simulink model "ES106A_StHlthSigStc"  (R2013b)
settings: Solver=FixedStepDiscrete  SolverMode=SingleTasking  StartTime=0.0  StopTime=1  FixedStep=0.002  RelTol=1e-3
undefined symbols (not defined in the file): APPL10_CNT_U08, BITSPERBYTE_CNT_U08, ENOTOK_CNT_U08, EOK_CNT_U08, LOWRMASKVAL_CNT_U32, NROFCRCAREA_CNT_U08, NVMAVRGPOSN_CNT_U08, NvmGetErrSts1, NVMMAXPOSN_CNT_U08, NVMMINPOSN_CNT_U08, NVMSAMPLECNTRPOSN_CNT_U08, RAMMAXPOSN_CNT_U08, RAMMINPOSN_CNT_U08, RAMRAWPOSN_CNT_U08, SIGCNT_ULS_U08, SigStcPrmInst, STHLTHMAXVAL_CNT_U08, STHLTHOSAPPL_CNT_U16, StHlthTaskRef1, WORDSIZE_CNT_U08
libraries: simulink x43, NxtrNvM x4, NxtrMax x4, NxtrMin x4, FloatToFixd x3, NxtrLim x2
(part 5 of 5)

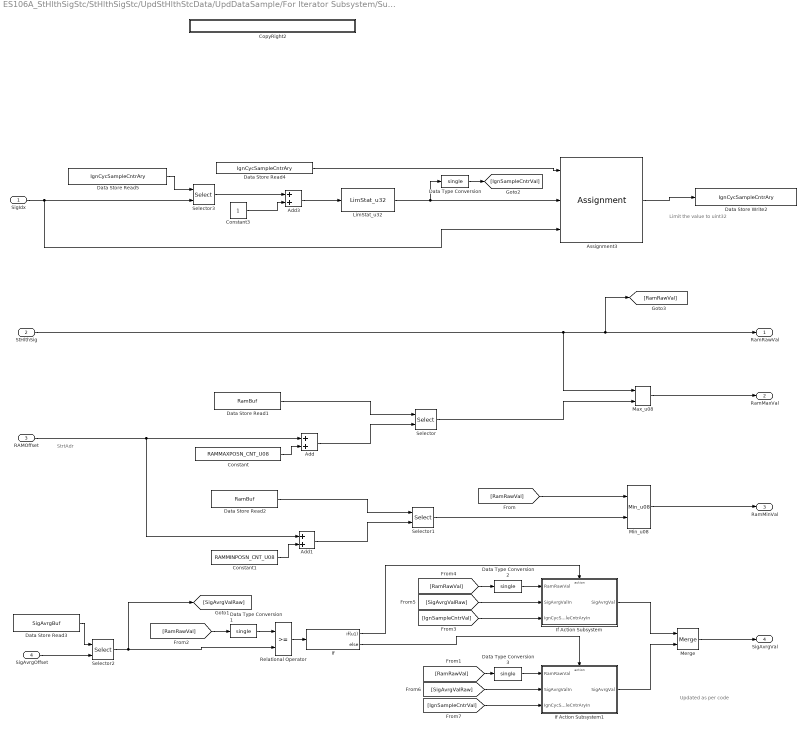
== system ES106A_StHlthSigStc/StHlthSigStc/UpdStHlthStcData/UpdDataSample/For Iterator Subsystem/Subsystem2/If Action Subsystem ==
  note: Updated as per code
  note: StrtAdr
  note: Limit the value to uint32
  SigIdx : Inport
  StHlthSig : Inport  Port=2
  RAMOffset : Inport  Port=3
  SigAvrgOffset : Inport  Port=4
  Add : Sum
  Add1 : Sum
  Add3 : Sum
  Assignment3 : Assignment  IndexMode=Zero-based  IndexOptions=Starting index (port)  Indices=1  OutputSizes=1
  Constant : Constant  Value=RAMMAXPOSN_CNT_U08  OutDataTypeStr=uint8
      settings: AttributesFormatString=%<OutDataTypeStr>
  Constant1 : Constant  Value=RAMMINPOSN_CNT_U08  OutDataTypeStr=uint8
      settings: AttributesFormatString=%<OutDataTypeStr>
  Constant3 : Constant  OutDataTypeStr=uint8
      settings: AttributesFormatString=%<OutDataTypeStr>
  CopyRight2 : Subsystem  Description=|  mask(Copyright Information){none=on}
      | Copyright info block.                                               
      |                                                                     
      | Place copyright information at the top of every subsystem in design.
      mask prompts: none "No parameters"
      mask help: Place copyright information at the top of every subsystem in design.
      mask Display:
      | NxtrConf = 'Nexteer Confidential';
      | 
      | sys = bdroot; %handle for the current model ("system")
      | first = get_param(sys,'Created');
      | first = first(end-3:end);  %year is last four digits
      | 
      | last = get_param(sys,'LastModifiedDate');
      | if isempty(last)
      |     last = datestr(now,'yyyy');
      | else
      |     last = last(end-3:end);
      | end
      | 
      | if strcmp(first,last)
      |     fprintf('%s -- Copyright %s Nexteer',NxtrConf,first)
      | else
      |     fprintf('%s -- %s%s- %s Nexteer',NxtrConf,char(169),first,last)
      | end
  Data Store Read1 : DataStoreRead  DataStoreName=RamBuf
  Data Store Read2 : DataStoreRead  DataStoreName=RamBuf
  Data Store Read3 : DataStoreRead  DataStoreName=SigAvrgBuf
  Data Store Read4 : DataStoreRead  Priority=2  DataStoreName=IgnCycSampleCntrAry
      settings: AttributesFormatString=Priority: %<Priority>
  Data Store Read5 : DataStoreRead  Priority=1  DataStoreName=IgnCycSampleCntrAry
      settings: AttributesFormatString=Priority: %<Priority>
  Data Store Write2 : DataStoreWrite  Priority=3  DataStoreName=IgnCycSampleCntrAry
      settings: AttributesFormatString=Priority: %<Priority>
  Data Type Conversion{,1..3} (4 alike) : DataTypeConversion  OutDataTypeStr=single
  If : If  IfExpression=u1
  If Action Subsystem : Subsystem  TreatAsAtomicUnit=on
  If Action Subsystem1 : Subsystem  TreatAsAtomicUnit=on
  LimStat_u32 : NxtrLim/LimStat_u32  LoLim=IGNCYCSAMPLECNTRARYMINLIM_CNT_U32  HiLim=IGNCYCSAMPLECNTRARYMAXLIM_CNT_U32
      settings: AttributesFormatString=|
      | Low Limit: %<LoLim>
      | High Limit:%<HiLim>
  Max_u08 : NxtrMax/Max_u08  SFunctionSpec="uint8 y1 = Max_u08( uint8 u1,  uint8 u2)"
      settings: AttributesFormatString=%<Name>
  Merge : Merge
  Min_u08 : NxtrMin/Min_u08  SFunctionSpec="uint8 y1 = Min_u08( uint8 u1,  uint8 u2)"  ShowSpec=off
      settings: AttributesFormatString=%<Name>
  Relational Operator : RelationalOperator  OutDataTypeStr=boolean
  Selector : Selector  IndexMode=Zero-based  InputPortWidth=66  IndexOptions=Starting index (port)  Indices=[1 3]  OutputSizes=1
  Selector1 : Selector  IndexMode=Zero-based  InputPortWidth=66  IndexOptions=Starting index (port)  Indices=[1 3]  OutputSizes=1
  Selector2 : Selector  IndexMode=Zero-based  InputPortWidth=22  IndexOptions=Starting index (port)  Indices=[1 3]  OutputSizes=1
  Selector3 : Selector  IndexMode=Zero-based  InputPortWidth=22  IndexOptions=Starting index (port)  Indices=[1 3]  OutputSizes=1
  RamRawVal : Outport
  RamMaxVal : Outport  Port=2
  RamMinVal : Outport  Port=3
  SigAvrgVal : Outport  Port=4
  wires:
  Data Store Read1/1 -> Selector/1
  Constant/1 -> Add/2
  Add/1 -> Selector/2
  Selector/1 -> Max_u08/2
  Data Store Read2/1 -> Selector1/1
  Constant1/1 -> Add1/2
  Add1/1 -> Selector1/2
  Selector1/1 -> Min_u08/2
  Data Store Read3/1 -> Selector2/1
  RAMOffset/1 -> Add1/1, Add/1
  Max_u08/1 -> RamMaxVal/1
  [RamRawVal] -> Min_u08/1
  Min_u08/1 -> RamMinVal/1
  Relational Operator/1 -> If/1
  If/1 -> If Action Subsystem/Action
  If/2 -> If Action Subsystem1/Action
  Merge/1 -> SigAvrgVal/1
  If Action Subsystem/1(SigAvrgVal) -> Merge/1
  If Action Subsystem1/1(SigAvrgVal) -> Merge/2
  [IgnSampleCntrVal] -> If Action Subsystem/3(IgnCycSampleCntrAryIn)
  SigAvrgOffset/1 -> Selector2/2
  [SigAvrgValRaw] -> If Action Subsystem1/2(SigAvrgValIn)
  [SigAvrgValRaw] -> If Action Subsystem/2(SigAvrgValIn)
  Selector2/1 -> Relational Operator/2, [SigAvrgValRaw]
  [RamRawVal] -> Data Type Conversion2/1
  [RamRawVal] -> Data Type Conversion3/1
  [RamRawVal] -> Data Type Conversion1/1
  Data Store Read5/1 -> Selector3/1
  Selector3/1 -> Add3/1
  Constant3/1 -> Add3/2
  Assignment3/1 -> Data Store Write2/1
  Add3/1 -> LimStat_u32/1
  Data Store Read4/1 -> Assignment3/1
  SigIdx/1 -> Assignment3/3, Selector3/2
  LimStat_u32/1 -> Data Type Conversion/1, Assignment3/2
  Data Type Conversion/1 -> [IgnSampleCntrVal]
  [IgnSampleCntrVal] -> If Action Subsystem1/3(IgnCycSampleCntrAryIn)
  StHlthSig/1 -> [RamRawVal], RamRawVal/1, Max_u08/1
  Data Type Conversion1/1 -> Relational Operator/1
  Data Type Conversion2/1 -> If Action Subsystem/1(RamRawVal)
  Data Type Conversion3/1 -> If Action Subsystem1/1(RamRawVal)

== system ES106A_StHlthSigStc/StHlthSigStc/UpdStHlthStcData/UpdDataSample/For Iterator Subsystem/Subsystem2/UpdateRamBuf ==
  note: RamAvrgVal Input was deleted
  RAMLocation : Inport
  RamRawVal : Inport  Port=2
  RamMaxVal : Inport  Port=3
  RamMinVal : Inport  Port=4
  Assignment4 : Assignment  IndexMode=Zero-based  IndexOptions=Starting index (port)  Indices=1  OutputSizes=1
  CopyRight2 : Subsystem  Description=|  mask(Copyright Information){none=on}
      | Copyright info block.                                               
      |                                                                     
      | Place copyright information at the top of every subsystem in design.
      mask prompts: none "No parameters"
      mask help: Place copyright information at the top of every subsystem in design.
      mask Display:
      | NxtrConf = 'Nexteer Confidential';
      | 
      | sys = bdroot; %handle for the current model ("system")
      | first = get_param(sys,'Created');
      | first = first(end-3:end);  %year is last four digits
      | 
      | last = get_param(sys,'LastModifiedDate');
      | if isempty(last)
      |     last = datestr(now,'yyyy');
      | else
      |     last = last(end-3:end);
      | end
      | 
      | if strcmp(first,last)
      |     fprintf('%s -- Copyright %s Nexteer',NxtrConf,first)
      | else
      |     fprintf('%s -- %s%s- %s Nexteer',NxtrConf,char(169),first,last)
      | end
  Data Store Read1 : DataStoreRead  DataStoreName=RamBuf
  Data Store Write2 : DataStoreWrite  DataStoreName=RamBuf
  Mux : Mux  Inputs=3
  wires:
  Data Store Read1/1 -> Assignment4/1
  RAMLocation/1 -> Assignment4/3
  Mux/1 -> Assignment4/2
  Assignment4/1 -> Data Store Write2/1
  RamRawVal/1 -> Mux/1
  RamMaxVal/1 -> Mux/2
  RamMinVal/1 -> Mux/3

== system ES106A_StHlthSigStc/StHlthSigStc/UpdStHlthStcData/UpdDataSample/For Iterator Subsystem/Subsystem2/UpdateSigAvrgBuf ==
  SigAvrgLocation : Inport
  SigAvrgVal : Inport  Port=2
  Assignment4 : Assignment  IndexMode=Zero-based  IndexOptions=Starting index (port)  Indices=1  OutputSizes=1
  CopyRight2 : Subsystem  Description=|  mask(Copyright Information){none=on}
      | Copyright info block.                                               
      |                                                                     
      | Place copyright information at the top of every subsystem in design.
      mask prompts: none "No parameters"
      mask help: Place copyright information at the top of every subsystem in design.
      mask Display:
      | NxtrConf = 'Nexteer Confidential';
      | 
      | sys = bdroot; %handle for the current model ("system")
      | first = get_param(sys,'Created');
      | first = first(end-3:end);  %year is last four digits
      | 
      | last = get_param(sys,'LastModifiedDate');
      | if isempty(last)
      |     last = datestr(now,'yyyy');
      | else
      |     last = last(end-3:end);
      | end
      | 
      | if strcmp(first,last)
      |     fprintf('%s -- Copyright %s Nexteer',NxtrConf,first)
      | else
      |     fprintf('%s -- %s%s- %s Nexteer',NxtrConf,char(169),first,last)
      | end
  Data Store Read1 : DataStoreRead  DataStoreName=SigAvrgBuf
  Data Store Write2 : DataStoreWrite  DataStoreName=SigAvrgBuf
  wires:
  Data Store Read1/1 -> Assignment4/1
  SigAvrgLocation/1 -> Assignment4/3
  Assignment4/1 -> Data Store Write2/1
  SigAvrgVal/1 -> Assignment4/2

== system ES106A_StHlthSigStc/StHlthSigStc/GetSigStcHlthData/If Action Subsystem1/GetSigStcHlthData/If Action Subsystem/While Iterator Subsystem/CopyRight2 ==

== system ES106A_StHlthSigStc/StHlthSigStc/GetSigStcHlthData/If Action Subsystem1/GetSigStcHlthData/If Action Subsystem/While Iterator Subsystem/Switch Case Action Subsystem ==
  In1 : Inport
  Action Port : ActionPort  ActionType=case
  CopyRight2 : Subsystem  Description=|  mask(Copyright Information){none=on}
      | Copyright info block.                                               
      |                                                                     
      | Place copyright information at the top of every subsystem in design.
      mask prompts: none "No parameters"
      mask help: Place copyright information at the top of every subsystem in design.
      mask Display:
      | NxtrConf = 'Nexteer Confidential';
      | 
      | sys = bdroot; %handle for the current model ("system")
      | first = get_param(sys,'Created');
      | if(isempty(first))
      |     first = datestr(now,'yyyy');
      | else
      |     first = first(end-3:end);  %year is last four digits
      | end
      | 
      | last = get_param(sys,'LastModifiedDate');
      | if isempty(last)
      |     last = datestr(now,'yyyy');
      | else
      |     last = last(end-3:end);
      | end
      | 
      | if strcmp(first,last)
      |     fprintf('%s -- Copyright %s Nexteer',NxtrConf,first)
      | else
      |     fprintf('%s -- %s%s- %s Nexteer',NxtrConf,char(169),first,last)
      | end
  Data Type Conversion : DataTypeConversion  OutDataTypeStr=uint32
  Shift Arithmetic3 : ArithShift  BitShiftNumber=SHIFTFAC24_ULS_U08  BitShiftDirection=Left
  Out1 : Outport
  wires:
  In1/1 -> Data Type Conversion/1
  Data Type Conversion/1 -> Shift Arithmetic3/1
  Shift Arithmetic3/1 -> Out1/1

== system ES106A_StHlthSigStc/StHlthSigStc/GetSigStcHlthData/If Action Subsystem1/GetSigStcHlthData/If Action Subsystem/While Iterator Subsystem/Switch Case Action Subsystem1 ==
  In1 : Inport
  Action Port : ActionPort  ActionType=case
  CopyRight2 : Subsystem  Description=|  mask(Copyright Information){none=on}
      | Copyright info block.                                               
      |                                                                     
      | Place copyright information at the top of every subsystem in design.
      mask prompts: none "No parameters"
      mask help: Place copyright information at the top of every subsystem in design.
      mask Display:
      | NxtrConf = 'Nexteer Confidential';
      | 
      | sys = bdroot; %handle for the current model ("system")
      | first = get_param(sys,'Created');
      | if(isempty(first))
      |     first = datestr(now,'yyyy');
      | else
      |     first = first(end-3:end);  %year is last four digits
      | end
      | 
      | last = get_param(sys,'LastModifiedDate');
      | if isempty(last)
      |     last = datestr(now,'yyyy');
      | else
      |     last = last(end-3:end);
      | end
      | 
      | if strcmp(first,last)
      |     fprintf('%s -- Copyright %s Nexteer',NxtrConf,first)
      | else
      |     fprintf('%s -- %s%s- %s Nexteer',NxtrConf,char(169),first,last)
      | end
  Data Type Conversion1 : DataTypeConversion  OutDataTypeStr=uint32
  Shift Arithmetic1 : ArithShift  BitShiftNumber=SHIFTFAC16_ULS_U08  BitShiftDirection=Left
  Out1 : Outport
  wires:
  In1/1 -> Data Type Conversion1/1
  Shift Arithmetic1/1 -> Out1/1
  Data Type Conversion1/1 -> Shift Arithmetic1/1

== system ES106A_StHlthSigStc/StHlthSigStc/GetSigStcHlthData/If Action Subsystem1/GetSigStcHlthData/If Action Subsystem/While Iterator Subsystem/Switch Case Action Subsystem2 ==
  In1 : Inport
  Action Port : ActionPort  ActionType=case
  CopyRight2 : Subsystem  Description=|  mask(Copyright Information){none=on}
      | Copyright info block.                                               
      |                                                                     
      | Place copyright information at the top of every subsystem in design.
      mask prompts: none "No parameters"
      mask help: Place copyright information at the top of every subsystem in design.
      mask Display:
      | NxtrConf = 'Nexteer Confidential';
      | 
      | sys = bdroot; %handle for the current model ("system")
      | first = get_param(sys,'Created');
      | if(isempty(first))
      |     first = datestr(now,'yyyy');
      | else
      |     first = first(end-3:end);  %year is last four digits
      | end
      | 
      | last = get_param(sys,'LastModifiedDate');
      | if isempty(last)
      |     last = datestr(now,'yyyy');
      | else
      |     last = last(end-3:end);
      | end
      | 
      | if strcmp(first,last)
      |     fprintf('%s -- Copyright %s Nexteer',NxtrConf,first)
      | else
      |     fprintf('%s -- %s%s- %s Nexteer',NxtrConf,char(169),first,last)
      | end
  Data Type Conversion1 : DataTypeConversion  OutDataTypeStr=uint32
  Shift Arithmetic2 : ArithShift  BitShiftNumber=SHIFTFAC8_ULS_U08  BitShiftDirection=Left
  Out1 : Outport
  wires:
  In1/1 -> Data Type Conversion1/1
  Data Type Conversion1/1 -> Shift Arithmetic2/1
  Shift Arithmetic2/1 -> Out1/1

== system ES106A_StHlthSigStc/StHlthSigStc/GetSigStcHlthData/If Action Subsystem1/GetSigStcHlthData/If Action Subsystem/While Iterator Subsystem/Switch Case Action Subsystem3 ==
  In1 : Inport
  Action Port : ActionPort  ActionType=case
  CopyRight2 : Subsystem  Description=|  mask(Copyright Information){none=on}
      | Copyright info block.                                               
      |                                                                     
      | Place copyright information at the top of every subsystem in design.
      mask prompts: none "No parameters"
      mask help: Place copyright information at the top of every subsystem in design.
      mask Display:
      | NxtrConf = 'Nexteer Confidential';
      | 
      | sys = bdroot; %handle for the current model ("system")
      | first = get_param(sys,'Created');
      | if(isempty(first))
      |     first = datestr(now,'yyyy');
      | else
      |     first = first(end-3:end);  %year is last four digits
      | end
      | 
      | last = get_param(sys,'LastModifiedDate');
      | if isempty(last)
      |     last = datestr(now,'yyyy');
      | else
      |     last = last(end-3:end);
      | end
      | 
      | if strcmp(first,last)
      |     fprintf('%s -- Copyright %s Nexteer',NxtrConf,first)
      | else
      |     fprintf('%s -- %s%s- %s Nexteer',NxtrConf,char(169),first,last)
      | end
  Data Type Conversion1 : DataTypeConversion  OutDataTypeStr=uint32
  Out1 : Outport
  wires:
  In1/1 -> Data Type Conversion1/1
  Data Type Conversion1/1 -> Out1/1

== system ES106A_StHlthSigStc/StHlthSigStc/StHlthStcPwrDwn/For Iterator Subsystem/If Action Subsystem/Statistical data computation for Controller Life Cycle/While Iterator Subsystem/CopyRight2 ==

== system ES106A_StHlthSigStc/StHlthSigStc/StHlthStcPwrDwn/For Iterator Subsystem/If Action Subsystem/Statistical data computation for Controller Life Cycle/While Iterator Subsystem/Switch Case Action Subsystem ==
  In1 : Inport
  Action Port : ActionPort  ActionType=case
  CopyRight2 : Subsystem  Description=|  mask(Copyright Information){none=on}
      | Copyright info block.                                               
      |                                                                     
      | Place copyright information at the top of every subsystem in design.
      mask prompts: none "No parameters"
      mask help: Place copyright information at the top of every subsystem in design.
      mask Display:
      | NxtrConf = 'Nexteer Confidential';
      | 
      | sys = bdroot; %handle for the current model ("system")
      | first = get_param(sys,'Created');
      | if(isempty(first))
      |     first = datestr(now,'yyyy');
      | else
      |     first = first(end-3:end);  %year is last four digits
      | end
      | 
      | last = get_param(sys,'LastModifiedDate');
      | if isempty(last)
      |     last = datestr(now,'yyyy');
      | else
      |     last = last(end-3:end);
      | end
      | 
      | if strcmp(first,last)
      |     fprintf('%s -- Copyright %s Nexteer',NxtrConf,first)
      | else
      |     fprintf('%s -- %s%s- %s Nexteer',NxtrConf,char(169),first,last)
      | end
  Data Type Conversion : DataTypeConversion  OutDataTypeStr=uint32
  Shift Arithmetic3 : ArithShift  BitShiftNumber=SHIFTFAC24_ULS_U08  BitShiftDirection=Left
  Out1 : Outport
  wires:
  In1/1 -> Data Type Conversion/1
  Data Type Conversion/1 -> Shift Arithmetic3/1
  Shift Arithmetic3/1 -> Out1/1

== system ES106A_StHlthSigStc/StHlthSigStc/StHlthStcPwrDwn/For Iterator Subsystem/If Action Subsystem/Statistical data computation for Controller Life Cycle/While Iterator Subsystem/Switch Case Action Subsystem1 ==
  In1 : Inport
  Action Port : ActionPort  ActionType=case
  CopyRight2 : Subsystem  Description=|  mask(Copyright Information){none=on}
      | Copyright info block.                                               
      |                                                                     
      | Place copyright information at the top of every subsystem in design.
      mask prompts: none "No parameters"
      mask help: Place copyright information at the top of every subsystem in design.
      mask Display:
      | NxtrConf = 'Nexteer Confidential';
      | 
      | sys = bdroot; %handle for the current model ("system")
      | first = get_param(sys,'Created');
      | if(isempty(first))
      |     first = datestr(now,'yyyy');
      | else
      |     first = first(end-3:end);  %year is last four digits
      | end
      | 
      | last = get_param(sys,'LastModifiedDate');
      | if isempty(last)
      |     last = datestr(now,'yyyy');
      | else
      |     last = last(end-3:end);
      | end
      | 
      | if strcmp(first,last)
      |     fprintf('%s -- Copyright %s Nexteer',NxtrConf,first)
      | else
      |     fprintf('%s -- %s%s- %s Nexteer',NxtrConf,char(169),first,last)
      | end
  Data Type Conversion1 : DataTypeConversion  OutDataTypeStr=uint32
  Shift Arithmetic1 : ArithShift  BitShiftNumber=SHIFTFAC16_ULS_U08  BitShiftDirection=Left
  Out1 : Outport
  wires:
  In1/1 -> Data Type Conversion1/1
  Shift Arithmetic1/1 -> Out1/1
  Data Type Conversion1/1 -> Shift Arithmetic1/1

== system ES106A_StHlthSigStc/StHlthSigStc/StHlthStcPwrDwn/For Iterator Subsystem/If Action Subsystem/Statistical data computation for Controller Life Cycle/While Iterator Subsystem/Switch Case Action Subsystem2 ==
  In1 : Inport
  Action Port : ActionPort  ActionType=case
  CopyRight2 : Subsystem  Description=|  mask(Copyright Information){none=on}
      | Copyright info block.                                               
      |                                                                     
      | Place copyright information at the top of every subsystem in design.
      mask prompts: none "No parameters"
      mask help: Place copyright information at the top of every subsystem in design.
      mask Display:
      | NxtrConf = 'Nexteer Confidential';
      | 
      | sys = bdroot; %handle for the current model ("system")
      | first = get_param(sys,'Created');
      | if(isempty(first))
      |     first = datestr(now,'yyyy');
      | else
      |     first = first(end-3:end);  %year is last four digits
      | end
      | 
      | last = get_param(sys,'LastModifiedDate');
      | if isempty(last)
      |     last = datestr(now,'yyyy');
      | else
      |     last = last(end-3:end);
      | end
      | 
      | if strcmp(first,last)
      |     fprintf('%s -- Copyright %s Nexteer',NxtrConf,first)
      | else
      |     fprintf('%s -- %s%s- %s Nexteer',NxtrConf,char(169),first,last)
      | end
  Data Type Conversion1 : DataTypeConversion  OutDataTypeStr=uint32
  Shift Arithmetic2 : ArithShift  BitShiftNumber=SHIFTFAC8_ULS_U08  BitShiftDirection=Left
  Out1 : Outport
  wires:
  In1/1 -> Data Type Conversion1/1
  Data Type Conversion1/1 -> Shift Arithmetic2/1
  Shift Arithmetic2/1 -> Out1/1

== system ES106A_StHlthSigStc/StHlthSigStc/StHlthStcPwrDwn/For Iterator Subsystem/If Action Subsystem/Statistical data computation for Controller Life Cycle/While Iterator Subsystem/Switch Case Action Subsystem3 ==
  In1 : Inport
  Action Port : ActionPort  ActionType=case
  CopyRight2 : Subsystem  Description=|  mask(Copyright Information){none=on}
      | Copyright info block.                                               
      |                                                                     
      | Place copyright information at the top of every subsystem in design.
      mask prompts: none "No parameters"
      mask help: Place copyright information at the top of every subsystem in design.
      mask Display:
      | NxtrConf = 'Nexteer Confidential';
      | 
      | sys = bdroot; %handle for the current model ("system")
      | first = get_param(sys,'Created');
      | if(isempty(first))
      |     first = datestr(now,'yyyy');
      | else
      |     first = first(end-3:end);  %year is last four digits
      | end
      | 
      | last = get_param(sys,'LastModifiedDate');
      | if isempty(last)
      |     last = datestr(now,'yyyy');
      | else
      |     last = last(end-3:end);
      | end
      | 
      | if strcmp(first,last)
      |     fprintf('%s -- Copyright %s Nexteer',NxtrConf,first)
      | else
      |     fprintf('%s -- %s%s- %s Nexteer',NxtrConf,char(169),first,last)
      | end
  Data Type Conversion1 : DataTypeConversion  OutDataTypeStr=uint32
  Out1 : Outport
  wires:
  In1/1 -> Data Type Conversion1/1
  Data Type Conversion1/1 -> Out1/1

== system ES106A_StHlthSigStc/StHlthSigStc/StHlthStcPwrDwn/For Iterator Subsystem/If Action Subsystem/Update Nvm/Subsystem/CopyRight2 ==

== system ES106A_StHlthSigStc/StHlthSigStc/StHlthStcPwrDwn/For Iterator Subsystem/If Action Subsystem/Update Nvm/Subsystem1/CopyRight2 ==

== system ES106A_StHlthSigStc/StHlthSigStc/UpdStHlthStcData/Call Non Trusted Function /For Iterator Subsystem/Subsystem2/If Action Subsystem/CopyRight2 ==

== system ES106A_StHlthSigStc/StHlthSigStc/UpdStHlthStcData/Call Non Trusted Function /For Iterator Subsystem/Subsystem2/If Action Subsystem/If Action Subsystem ==
  RamRawVal : Inport
  SigAvrgValIn : Inport  Port=2
  IgnCycSampleCntrAryIn : Inport  Port=3
  Action Port : ActionPort  ActionType=then
  Add1 : Sum
  Add4 : Sum  Inputs=+-
  Divide : Product  Inputs=*/
  SigAvrgVal : Outport
  wires:
  [SigAvrgVal] -> Add4/2
  RamRawVal/1 -> Add4/1
  Add4/1 -> Divide/1
  IgnCycSampleCntrAryIn/1 -> Divide/2
  SigAvrgValIn/1 -> [SigAvrgVal]
  Divide/1 -> Add1/2
  [SigAvrgVal] -> Add1/1
  Add1/1 -> SigAvrgVal/1

== system ES106A_StHlthSigStc/StHlthSigStc/UpdStHlthStcData/Call Non Trusted Function /For Iterator Subsystem/Subsystem2/If Action Subsystem/If Action Subsystem1 ==
  RamRawVal : Inport
  SigAvrgValIn : Inport  Port=2
  IgnCycSampleCntrAryIn : Inport  Port=3
  Action Port : ActionPort  ActionType=else
  Add1 : Sum  Inputs=+-
  Add4 : Sum  Inputs=+-
  Divide : Product  Inputs=*/
  SigAvrgVal : Outport
  wires:
  RamRawVal/1 -> Add4/2
  Add4/1 -> Divide/1
  IgnCycSampleCntrAryIn/1 -> Divide/2
  SigAvrgValIn/1 -> [SigAvrgVal]
  Divide/1 -> Add1/2
  [SigAvrgVal] -> Add1/1
  Add1/1 -> SigAvrgVal/1
  [SigAvrgVal] -> Add4/1

== system ES106A_StHlthSigStc/StHlthSigStc/UpdStHlthStcData/Call Non Trusted Function /For Iterator Subsystem/Subsystem2/UpdateRamBuf/CopyRight2 ==

== system ES106A_StHlthSigStc/StHlthSigStc/UpdStHlthStcData/Call Non Trusted Function /For Iterator Subsystem/Subsystem2/UpdateSigAvrgBuf/CopyRight2 ==

== system ES106A_StHlthSigStc/StHlthSigStc/UpdStHlthStcData/UpdDataSample/For Iterator Subsystem/Subsystem2/If Action Subsystem/CopyRight2 ==

== system ES106A_StHlthSigStc/StHlthSigStc/UpdStHlthStcData/UpdDataSample/For Iterator Subsystem/Subsystem2/If Action Subsystem/If Action Subsystem ==
  RamRawVal : Inport
  SigAvrgValIn : Inport  Port=2
  IgnCycSampleCntrAryIn : Inport  Port=3
  Action Port : ActionPort  ActionType=then
  Add1 : Sum
  Add4 : Sum  Inputs=+-
  Divide : Product  Inputs=*/
  SigAvrgVal : Outport
  wires:
  [SigAvrgVal] -> Add4/2
  RamRawVal/1 -> Add4/1
  Add4/1 -> Divide/1
  IgnCycSampleCntrAryIn/1 -> Divide/2
  SigAvrgValIn/1 -> [SigAvrgVal]
  Divide/1 -> Add1/2
  [SigAvrgVal] -> Add1/1
  Add1/1 -> SigAvrgVal/1

== system ES106A_StHlthSigStc/StHlthSigStc/UpdStHlthStcData/UpdDataSample/For Iterator Subsystem/Subsystem2/If Action Subsystem/If Action Subsystem1 ==
  RamRawVal : Inport
  SigAvrgValIn : Inport  Port=2
  IgnCycSampleCntrAryIn : Inport  Port=3
  Action Port : ActionPort  ActionType=else
  Add1 : Sum  Inputs=+-
  Add4 : Sum  Inputs=+-
  Divide : Product  Inputs=*/
  SigAvrgVal : Outport
  wires:
  RamRawVal/1 -> Add4/2
  Add4/1 -> Divide/1
  IgnCycSampleCntrAryIn/1 -> Divide/2
  SigAvrgValIn/1 -> [SigAvrgVal]
  Divide/1 -> Add1/2
  [SigAvrgVal] -> Add1/1
  Add1/1 -> SigAvrgVal/1
  [SigAvrgVal] -> Add4/1

== system ES106A_StHlthSigStc/StHlthSigStc/UpdStHlthStcData/UpdDataSample/For Iterator Subsystem/Subsystem2/UpdateRamBuf/CopyRight2 ==

== system ES106A_StHlthSigStc/StHlthSigStc/UpdStHlthStcData/UpdDataSample/For Iterator Subsystem/Subsystem2/UpdateSigAvrgBuf/CopyRight2 ==

== system ES106A_StHlthSigStc/StHlthSigStc/GetSigStcHlthData/If Action Subsystem1/GetSigStcHlthData/If Action Subsystem/While Iterator Subsystem/Switch Case Action Subsystem/CopyRight2 ==

== system ES106A_StHlthSigStc/StHlthSigStc/GetSigStcHlthData/If Action Subsystem1/GetSigStcHlthData/If Action Subsystem/While Iterator Subsystem/Switch Case Action Subsystem1/CopyRight2 ==

== system ES106A_StHlthSigStc/StHlthSigStc/GetSigStcHlthData/If Action Subsystem1/GetSigStcHlthData/If Action Subsystem/While Iterator Subsystem/Switch Case Action Subsystem2/CopyRight2 ==

== system ES106A_StHlthSigStc/StHlthSigStc/GetSigStcHlthData/If Action Subsystem1/GetSigStcHlthData/If Action Subsystem/While Iterator Subsystem/Switch Case Action Subsystem3/CopyRight2 ==

== system ES106A_StHlthSigStc/StHlthSigStc/StHlthStcPwrDwn/For Iterator Subsystem/If Action Subsystem/Statistical data computation for Controller Life Cycle/While Iterator Subsystem/Switch Case Action Subsystem/CopyRight2 ==

== system ES106A_StHlthSigStc/StHlthSigStc/StHlthStcPwrDwn/For Iterator Subsystem/If Action Subsystem/Statistical data computation for Controller Life Cycle/While Iterator Subsystem/Switch Case Action Subsystem1/CopyRight2 ==

== system ES106A_StHlthSigStc/StHlthSigStc/StHlthStcPwrDwn/For Iterator Subsystem/If Action Subsystem/Statistical data computation for Controller Life Cycle/While Iterator Subsystem/Switch Case Action Subsystem2/CopyRight2 ==

== system ES106A_StHlthSigStc/StHlthSigStc/StHlthStcPwrDwn/For Iterator Subsystem/If Action Subsystem/Statistical data computation for Controller Life Cycle/While Iterator Subsystem/Switch Case Action Subsystem3/CopyRight2 ==
